simulink model "sim_IMP_LQR_2018_2"  (R2018a)
settings: Solver=ode1  StartTime=0.0  StopTime=30  FixedStep=0.002  RelTol=1e-3  EnableMultiTasking=on
values from neighbouring files (symbols this model uses):
  A = [0 0 1 0 ... (first row only)    [IMP_LQR_Design_2.m]    (also in IMP_LQR_Design_C.m; IMP_LQR_Design_SepPrinc.m; IMP_LQR_Design_Seperation.m; IMP_LQR_Design_Seperation_Compare.m)
  A_aug = [A B*Cref; zeros(4,4) Aref]    [IMP_LQR_Design_2.m]    (also in IMP_LQR_Design_C.m; IMP_LQR_Design_SepPrinc.m; IMP_LQR_Design_Seperation.m; IMP_LQR_Design_Seperation_Compare.m)
  B = [0 0; 0 0; Kpp/Jp Kpy/Jp; Kyp/Jy Kyy/Jy]    [IMP_LQR_Design_2.m]    (also in IMP_LQR_Design_C.m; IMP_LQR_Design_SepPrinc.m; IMP_LQR_Design_Seperation.m; IMP_LQR_Design_Seperation_Compare.m)
  B_aug = [B; zeros(4,2)]    [IMP_LQR_Design_2.m]    (also in IMP_LQR_Design_C.m; IMP_LQR_Design_SepPrinc.m; IMP_LQR_Design_Seperation.m; IMP_LQR_Design_Seperation_Compare.m)
  C = [1 0 0 0; 0 1 0 0]    [IMP_LQR_Design_2.m]    (also in IMP_LQR_Design_C.m; IMP_LQR_Design_SepPrinc.m = [0 0 1 0; 0 1 0 0]; IMP_LQR_Design_Seperation.m; IMP_LQR_Design_Seperation_Compare.m = [0 1 0 0; 0 1 0 0])
  C_aug = [C zeros(2,4)]    [IMP_LQR_Design_2.m]    (also in IMP_LQR_Design_C.m; IMP_LQR_Design_SepPrinc.m; IMP_LQR_Design_Seperation.m; IMP_LQR_Design_Seperation_Compare.m)
  D = [0 0; 0 0]    [IMP_LQR_Design_2.m]    (also in IMP_LQR_Design_C.m; IMP_LQR_Design_SepPrinc.m; IMP_LQR_Design_Seperation.m; IMP_LQR_Design_Seperation_Compare.m)
  J = [J;J]    [IMP_LQR_Design_2.m]    (also in IMP_LQR_Design_C.m; IMP_LQR_Design_Seperation.m = J'; IMP_LQR_Design_Seperation_Compare.m = J'; design_C.m = place(A',C', polesj)')
  K = [K Cref]    [IMP_LQR_Design_2.m]    (also in IMP_LQR_Design_C.m; IMP_LQR_Design_SepPrinc.m; IMP_LQR_Design_Seperation.m; IMP_LQR_Design_Seperation_Compare.m)
  N = K(1:2,1:2)    [IMP_LQR_Design_2.m]    (also in IMP_LQR_Design_C.m; IMP_LQR_Design_SepPrinc.m; IMP_LQR_Design_Seperation.m; IMP_LQR_Design_Seperation_Compare.m)
libraries: simulink_extras x4
settings Model: ExtModeTrigDuration=5000  Creator=MLevis  LastModifiedBy=cdr_3
settings SolverCC: PositivePriorityOrder=on
settings DataIOCC: LimitDataPoints=on  SaveFormat=Array
settings OptimizationCC: LifeSpan=inf
settings DebuggingCC: SolverPrmCheckMsg=warning  SFUnexpectedBacktrackingDiag=warning  SFNoUnconditionalDefaultTransitionDiag=warning  SFExecutionAtInitializationDiag=none
settings HardwareCC: ProdBitPerPointer=32  ProdBitPerSizeT=32  ProdBitPerPtrDiffT=32  ProdLargestAtomicFloat=None  ProdIntDivRoundTo=Undefined  ProdEndianess=Unspecified  ProdWordSize=32  ProdHWDeviceType=32-bit Generic
settings ModelReferenceCC: PropagateSignalLabelsOutOfModel=off
settings RTWCC: SystemTargetFile=quarc_win64.tlc  TemplateMakefile=quarc_default_tmf  Description=QUARC Win64 Target
settings CodeAppCC: StateflowObjectComments=on
settings STFCustomTargetCC: TargetPreCompLibLocation=C:\PROGRA~3\QUARC\lib\2014a\win64\release  ConcurrentExecutionCompliant=on  GeneratePreprocessorConditionals=Disable all  SystemTargetFile=quarc_win64.tlc
settings GRTTargetCC: TargetPreCompLibLocation=C:\PROGRA~3\QUARC\lib\2014a\win64\release  TargetLangStandard=C89/C90 (ANSI)  ParMdlRefBuildCompliant=off  CompOptLevelCompliant=off  GeneratePreprocessorConditionals=Disable all  CombineOutputUpdateFcns=off  MatFileLogging=off  CPPClassGenCompliant=off  GRTInterface=on  UseToolchainInfoCompliant=off  ExtMode=on  ExtModeMexFile=quarc_comm
settings ConfigComp: CovMetricSettings=dw  CovHtmlReporting=on  CovSaveCumulativeToWorkspaceVar=on  CovSaveSingleToWorkspaceVar=on  CovExternalEMLEnable=off  CovSFcnEnable=off

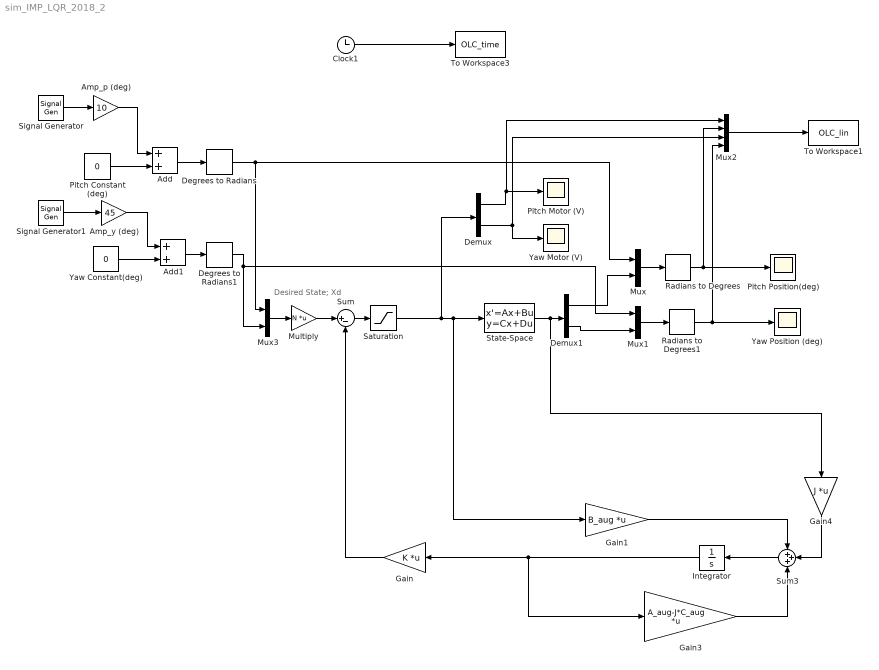
== system sim_IMP_LQR_2018_2 ==
  note: Desired State; Xd
  Add : Sum
  Add1 : Sum
  Amp_p (deg) : Gain  Gain=10
  Amp_y (deg) : Gain  Gain=45
  Clock1 : Clock
  Degrees to Radians : simulink_extras/Transformations/Degrees to Radians
  Degrees to Radians1 : simulink_extras/Transformations/Degrees to Radians
  Demux : Demux  Outputs=2
  Demux1 : Demux  Outputs=2
  Gain : Gain  Gain=K  Multiplication=Matrix(K*u)
  Gain1 : Gain  Gain=B_aug  Multiplication=Matrix(K*u)
  Gain3 : Gain  Gain=A_aug-J*C_aug  Multiplication=Matrix(K*u)
  Gain4 : Gain  Gain=J  Multiplication=Matrix(K*u)
  Integrator : Integrator
  Multiply : Gain  Gain=N  Multiplication=Matrix(K*u)
  Mux : Mux  Inputs=2
  Mux1 : Mux  Inputs=2
  Mux2 : Mux
  Mux3 : Mux  Inputs=2
  Pitch Constant (deg) : Constant  Value=0
  Pitch Motor (V) : Scope
  Pitch Position(deg) : Scope
  Radians to Degrees : simulink_extras/Transformations/Radians to Degrees
  Radians to Degrees1 : simulink_extras/Transformations/Radians to Degrees
  Saturation : Saturate  UpperLimit=24  LowerLimit=-24
  Signal Generator : SignalGenerator  Frequency=1/5
  Signal Generator1 : SignalGenerator  Frequency=1/10
  State-Space : StateSpace  A=A  B=B  C=C  D=D  InitialCondition=0
  Sum : Sum  Inputs=|+-
  Sum3 : Sum  Inputs=+++
  To Workspace1 : ToWorkspace  VariableName=OLC_lin  SampleTime=-1
  To Workspace3 : ToWorkspace  VariableName=OLC_time  SampleTime=-1
  Yaw Constant(deg) : Constant  Value=0
  Yaw Motor (V) : Scope
  Yaw Position (deg) : Scope
  wires:
  Degrees to Radians/1 -> Mux3/1, Mux/1
  Degrees to Radians1/1 -> Mux3/2, Mux1/1
  Signal Generator/1 -> Amp_p (deg)/1
  Pitch Constant (deg)/1 -> Add/2
  Add/1 -> Degrees to Radians/1
  Yaw Constant(deg)/1 -> Add1/2
  Amp_p (deg)/1 -> Add/1
  Signal Generator1/1 -> Amp_y (deg)/1
  Amp_y (deg)/1 -> Add1/1
  Add1/1 -> Degrees to Radians1/1
  Mux/1 -> Radians to Degrees/1
  Radians to Degrees/1 -> Mux2/2, Pitch Position(deg)/1
  Radians to Degrees1/1 -> Mux2/4, Yaw Position (deg)/1
  Demux/1 -> Mux2/1, Pitch Motor (V)/1
  Demux/2 -> Yaw Motor (V)/1, Mux2/3
  Mux1/1 -> Radians to Degrees1/1
  Mux3/1 -> Multiply/1
  Demux1/1 -> Mux/2
  Demux1/2 -> Mux1/2
  Sum/1 -> Saturation/1
  Gain1/1 -> Sum3/1
  Clock1/1 -> To Workspace3/1
  Mux2/1 -> To Workspace1/1
  State-Space/1 -> Gain4/1, Demux1/1
  Gain4/1 -> Sum3/2
  Gain3/1 -> Sum3/3
  Sum3/1 -> Integrator/1
  Integrator/1 -> Gain3/1, Gain/1
  Gain/1 -> Sum/2
  Saturation/1 -> Gain1/1, State-Space/1, Demux/1
  Multiply/1 -> Sum/1
